simulink model "sgMdl_IO753_IO754_ModbusTCP_Loopback"  (R2024b)
settings: Solver=FixedStepAuto  StartTime=0.0  StopTime=inf  RelTol=1e-3  EnableMultiTasking=on
undefined symbols (not defined in the file): C, IO, Mode, receive_v2, send_v2, setup_v2
libraries: slrealtimeutilitieslib x9, speedgoatlib_IO753 x4, speedgoatlib_IO754 x3, simulink x2
Description:
  | IO753 & IO754 - Modbus TCP Loopback
settings Model: sg_rtwmakecfg_data=_sg_IO75X_v1_2_0__sg_netxLib_MSVC140_  ModifiedByFormat=Speedgoat  SimulationMode=external  ExtModeTrigDuration=100000  Creator=Speedgoat  LastModifiedBy=Speedgoat
settings SolverCC: ConcurrentTasks=on  AlgebraicLoopSolver=TrustRegion  PositivePriorityOrder=on  AutoInsertRateTranBlk=on  InsertRTBMode=Never (minimum delay)
settings DataIOCC: LimitDataPoints=on  SaveFormat=StructureWithTime  ReturnWorkspaceOutputs=off
settings OptimizationCC: BlockReduction=off  BooleanDataType=off  OptimizeBlockIOStorage=off  BufferReuse=off  GlobalBufferReuse=off  ExpressionFolding=off  LocalBlockOutputs=off  OptimizeDataStoreBuffers=off  BusAssignmentInplaceUpdate=off
settings DebuggingCC: SaveWithParameterizedLinksMsg=none  UnderspecifiedInitializationDetection=Classic  MergeDetectMultiDrivingBlocksExec=none  SignalResolutionControl=TryResolveAllWithWarning  InheritedTsInSrcMsg=none  TasksWithSamePriorityMsg=none  ParameterOverflowMsg=none  UnconnectedInputMsg=warning  UnconnectedOutputMsg=warning  UnconnectedLineMsg=warning  SFUnexpectedBacktrackingDiag=warning  SFNoUnconditionalDefaultTransitionDiag=warning  SFExecutionAtInitializationDiag=none  ArithmeticOperatorsInVariantConditions=warning
settings HardwareCC: ProdBitPerLong=64  ProdLongLongMode=on  ProdHWDeviceType=Intel->x86-64 (Linux 64)  TargetBitPerPointer=64  TargetBitPerSizeT=64  TargetBitPerPtrDiffT=64  TargetLongLongMode=on  TargetIntDivRoundTo=Zero  TargetEndianess=LittleEndian  TargetWordSize=64  TargetHWDeviceType=MATLAB Host
settings ModelReferenceCC: EnableRefExpFcnMdlSchedulingChecks=on  PropagateSignalLabelsOutOfModel=off
settings SFSimCC: SimUseLocalCustomCode=off  CustomCodeUndefinedFunction=UseInterfaceOnly
settings RTWCC: Description=Speedgoat Real-Time Target Machine  SystemTargetFile=speedgoat.tlc  TemplateMakefile=slrealtime_default_tmf  RetainRTWFile=on  RTWUseLocalCustomCode=off  Toolchain=Simulink Real-Time Toolchain  BuildConfiguration=Faster Runs  TargetLang=C++  GPUComputeCapability=3.5  DLArmComputeVersion=19.05
settings CodeAppCC: StateflowObjectComments=on
settings SimulinkRealTimeTargetCC: SubcomponentCodeInterfacePackaging=Reusable function  InstructionSetFMA=off  LogToMDFFile=off  SLRTFileLogMaxRuns=10  UseGCCFastMath=on
settings ConfigComp: CovMetricSettings=dw  CovSaveCumulativeToWorkspaceVar=on  CovSaveSingleToWorkspaceVar=on  CovExternalEMLEnable=off  CovBoundaryAbsTol=1.0e-5

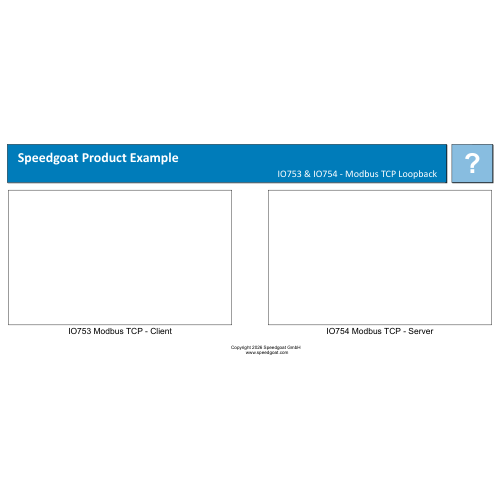
[thumbnail: Simulink's stored preview of the top-level diagram]
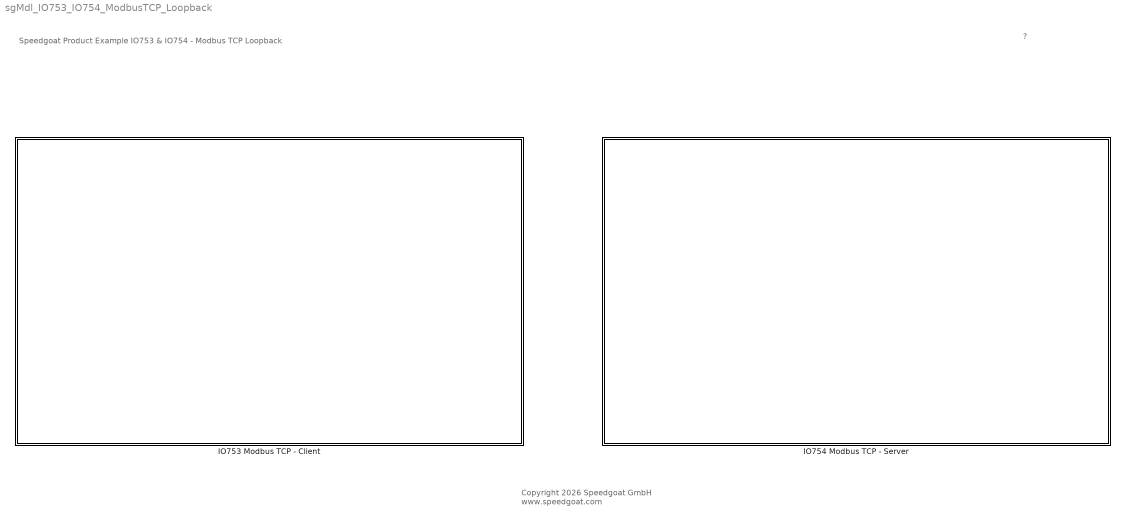
== system sgMdl_IO753_IO754_ModbusTCP_Loopback ==
  note: Speedgoat Product Example
      | IO753 & IO754 - Modbus TCP Loopback
  note: ?
  note: Copyright 2026 Speedgoat GmbH
      |  www.speedgoat.com
  IO753 Modbus TCP - Client : Subsystem
  IO754 Modbus TCP - Server : Subsystem

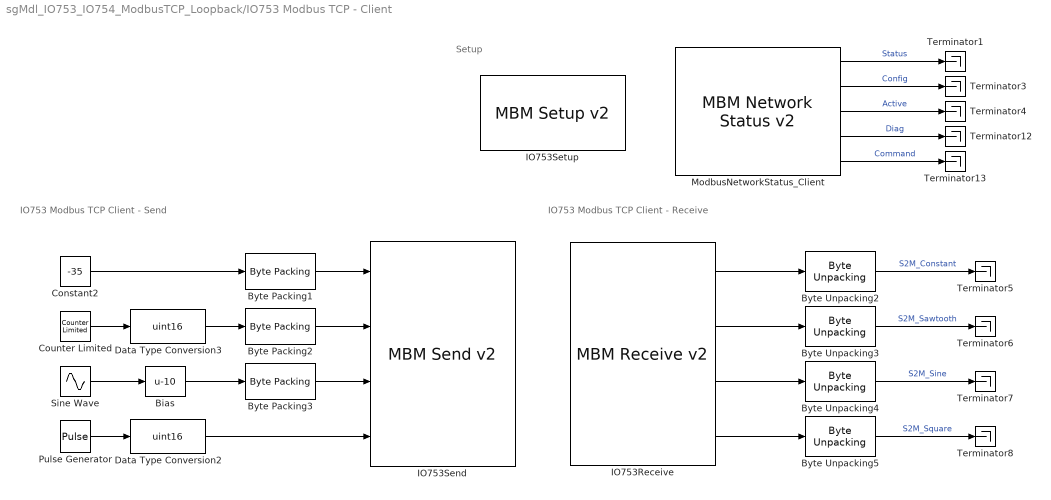
== system sgMdl_IO753_IO754_ModbusTCP_Loopback/IO753 Modbus TCP - Client ==
  note: IO753 Modbus TCP Client - Receive
  note: IO753 Modbus TCP Client - Send
  note: Setup
  Bias : Bias  Bias=-10
  Byte Packing1 : slrealtimeutilitieslib/Byte Packing  MaskPackedDataType=uint16  MaskUnpackedDataTypes={'double'}  MaskAlignment=1
  Byte Packing2 : slrealtimeutilitieslib/Byte Packing  MaskPackedDataType=uint16  MaskUnpackedDataTypes={'uint16'}  MaskAlignment=1
  Byte Packing3 : slrealtimeutilitieslib/Byte Packing  MaskPackedDataType=uint16  MaskUnpackedDataTypes={'double'}  MaskAlignment=1
  Byte Unpacking{2..5} (4 alike) : slrealtimeutilitieslib/Byte Unpacking
  Constant2 : Constant  Value=-35  SampleTime=-1
  Counter Limited : simulink/Sources/Counter Limited  uplimit=53  tsamp=-1
  Data Type Conversion2 : DataTypeConversion  OutMin=[0]  OutMax=[50]  OutDataTypeStr=uint16  SaturateOnIntegerOverflow=off  RndMeth=Floor
  Data Type Conversion3 : DataTypeConversion  OutMin=[0]  OutMax=[100]  OutDataTypeStr=uint16  SaturateOnIntegerOverflow=off  RndMeth=Floor
  IO753Receive : speedgoatlib_IO753/MBM Receive v2  id=1  parSampleTime=-1  parCommandTable={ 'Tx_Constant', 'IP_Server_00', '0', 'FC16 Write Multiple Registers', '0', '4', '50'; 'Tx_Sawtooth', 'IP_Server_00', '0', 'FC6 Write Single Register ', '4', '1', '50'; 'Tx_Sine', 'IP_Server_00', '0', 'FC16 Write Multiple Registers', '5', '4', '50'; 'Tx_Square', 'IP_Server_00', '0', 'FC16 Write Multiple Registers', '9', '1', '50'; 'Rx_Constant', 'IP_Server_00', '0', 'FC3 Read Holding Registers', '0', '1', '50'; 'Rx_Sawtooth', 'IP_Server_00', '0', 'FC3 Read Holding Registers', '1', '1', '50'; 'Rx_Sine', 'IP_Server_00', '0', 'FC3 Read Holding Registers', '2', '4', '50'; 'Rx_Square', 'IP_Server_00', '0', 'FC3 Read Holding Registers', '6', '1', '50' }
      settings: SourceProductName=Simulink Real-Time: Speedgoat I/O Blockset
  IO753Send : speedgoatlib_IO753/MBM Send v2  id=1  parSampleTime=-1  parCommandTable={ 'Tx_Constant', 'IP_Server_00', '0', 'FC16 Write Multiple Registers', '0', '4', '50'; 'Tx_Sawtooth', 'IP_Server_00', '0', 'FC6 Write Single Register ', '4', '1', '50'; 'Tx_Sine', 'IP_Server_00', '0', 'FC16 Write Multiple Registers', '5', '4', '50'; 'Tx_Square', 'IP_Server_00', '0', 'FC16 Write Multiple Registers', '9', '1', '50'; 'Rx_Constant', 'IP_Server_00', '0', 'FC3 Read Holding Registers', '0', '1', '50'; 'Rx_Sawtooth', 'IP_Server_00', '0', 'FC3 Read Holding Registers', '1', '1', '50'; 'Rx_Sine', 'IP_Server_00', '0', 'FC3 Read Holding Registers', '2', '4', '50'; 'Rx_Square', 'IP_Server_00', '0', 'FC3 Read Holding Registers', '6', '1', '50' }
      settings: SourceProductName=Simulink Real-Time: Speedgoat I/O Blockset
  IO753Setup : speedgoatlib_IO753/MBM Setup v2  id=1  parSlot=-1  parBusStart=Automatic  parIpAddress=IP_Client_00  parNetmask='255.255.255.0'  parGateway='0.0.0.0'  parBootP=off  parDHCP=off  DataSwap=off  parDelay=0  parCommandTable={ 'Tx_Constant', 'IP_Server_00', '0', 'FC16 Write Multiple Registers', '0', '4', '50'; 'Tx_Sawtooth', 'IP_Server_00', '0', 'FC6 Write Single Register ', '4', '1', '50'; 'Tx_Sine', 'IP_Server_00', '0', 'FC16 Write Multiple Registers', '5', '4', '50'; 'Tx_Square', 'IP_Server_00', '0', 'FC16 Write Multiple Registers', '9', '1', '50'; 'Rx_Constant', 'IP_Server_00', '0', 'FC3 Read Holding Registers', '0', '1', '50'; 'Rx_Sawtooth', 'IP_Server_00', '0', 'FC3 Read Holding Registers', '1', '1', '50'; 'Rx_Sine', 'IP_Server_00', '0', 'FC3 Read Holding Registers', '2', '4', '50'; 'Rx_Square', 'IP_Server_00', '0', 'FC3 Read Holding Registers', '6', '1', '50' }
      settings: SourceProductName=Simulink Real-Time: Speedgoat I/O Blockset
  ModbusNetworkStatus_Client : speedgoatlib_IO753/MBM Network Status v2  id=1  parSampleTime=-1  parSetStatus=off  parNumServers=0  parNumCommands=0
      settings: SourceProductName=Simulink Real-Time: Speedgoat I/O Blockset
  Pulse Generator : DiscretePulseGenerator  PulseType=Time based  Amplitude=23  Period=3.5  PulseWidth=40  SampleTime=-1
  Sine Wave : Sin  Amplitude=12  Frequency=pi  Phase=pi
  Terminator{1,3..8,12..13} (9 alike) : Terminator
  wires:
  Byte Unpacking4/1 -> Terminator7/1  "S2M_Sine"
  Sine Wave/1 -> Bias/1
  Pulse Generator/1 -> Data Type Conversion2/1
  Byte Unpacking3/1 -> Terminator6/1  "S2M_Sawtooth"
  Byte Unpacking5/1 -> Terminator8/1  "S2M_Square"
  Byte Unpacking2/1 -> Terminator5/1  "S2M_Constant"
  Counter Limited/1 -> Data Type Conversion3/1
  Byte Packing1/1 -> IO753Send/1
  Byte Packing2/1 -> IO753Send/2
  Byte Packing3/1 -> IO753Send/3
  Data Type Conversion2/1 -> IO753Send/4
  IO753Receive/1 -> Byte Unpacking2/1
  IO753Receive/2 -> Byte Unpacking3/1
  IO753Receive/3 -> Byte Unpacking4/1
  IO753Receive/4 -> Byte Unpacking5/1
  ModbusNetworkStatus_Client/2 -> Terminator3/1  "Config"
  ModbusNetworkStatus_Client/1 -> Terminator1/1  "Status"
  ModbusNetworkStatus_Client/3 -> Terminator4/1  "Active"
  ModbusNetworkStatus_Client/4 -> Terminator12/1  "Diag"
  ModbusNetworkStatus_Client/5 -> Terminator13/1  "Command"
  Data Type Conversion3/1 -> Byte Packing2/1
  Bias/1 -> Byte Packing3/1
  Constant2/1 -> Byte Packing1/1

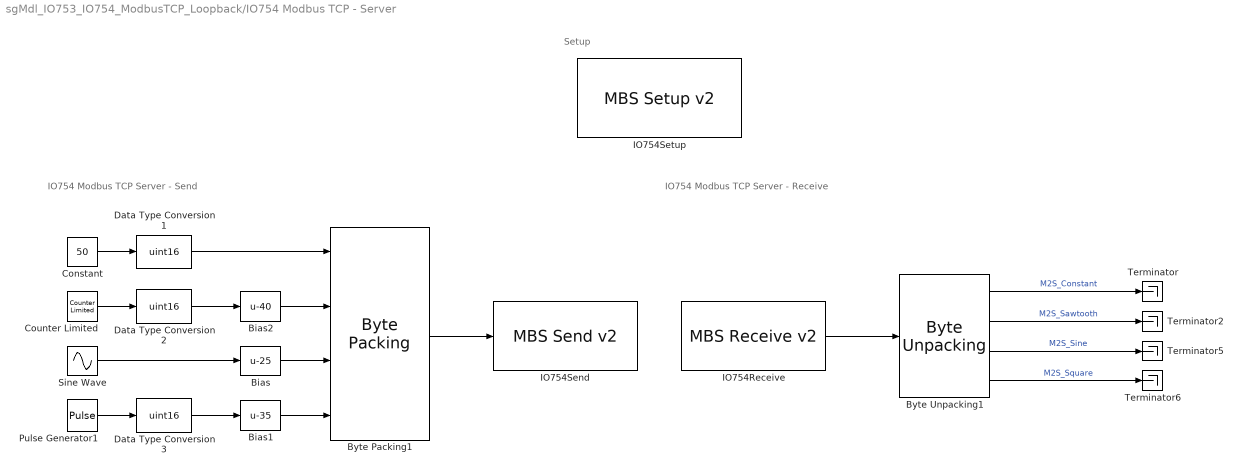
== system sgMdl_IO753_IO754_ModbusTCP_Loopback/IO754 Modbus TCP - Server ==
  note: Setup
  note: IO754 Modbus TCP Server - Send
  note: IO754 Modbus TCP Server - Receive
  Bias : Bias  Bias=-25  SaturateOnIntegerOverflow=off
  Bias1 : Bias  Bias=-35  SaturateOnIntegerOverflow=off
  Bias2 : Bias  Bias=-40  SaturateOnIntegerOverflow=off
  Byte Packing1 : slrealtimeutilitieslib/Byte Packing  MaskPackedDataType=uint8  MaskUnpackedDataTypes={'uint16','uint16','double','uint16'}  MaskAlignment=1
  Byte Unpacking1 : slrealtimeutilitieslib/Byte Unpacking  MaskUnpackedDataTypes={'double','uint16','double','uint16'}  MaskUnpackedDataSizes={[1],[1],[1],[1]}  MaskAlignment=1
  Constant : Constant  Value=50  OutDataTypeStr=Inherit: Inherit via back propagation  SampleTime=-1
  Counter Limited : simulink/Sources/Counter Limited  uplimit=42  tsamp=-1
  Data Type Conversion1 : DataTypeConversion  OutMin=[0]  OutMax=[100]  OutDataTypeStr=uint16  SaturateOnIntegerOverflow=off  RndMeth=Floor
  Data Type Conversion2 : DataTypeConversion  OutMin=[0]  OutMax=[100]  OutDataTypeStr=uint16  SaturateOnIntegerOverflow=off  RndMeth=Floor
  Data Type Conversion3 : DataTypeConversion  OutMin=[0]  OutMax=[50]  OutDataTypeStr=uint16  SaturateOnIntegerOverflow=off  RndMeth=Floor
  IO754Receive : speedgoatlib_IO754/IO-Mode/MBS Receive v2   id=2  portType=1 Port with n element vector of type UINT8  portDataBytes=20  sampleTime=-1  blockInfo=receive_v2;setup_v2  isSender=0  speedgoatMainProtl=IO75X_IO64X  speedgoatSubProtl=IO754
      settings: SourceProductName=Simulink Real-Time: Speedgoat I/O Blockset
  IO754Send : speedgoatlib_IO754/IO-Mode/MBS Send v2   id=2  portType=1 Port with n element vector of type UINT8  portDataBytes=14  sampleTime=-1  blockInfo=send_v2;setup_v2  isSender=1  speedgoatMainProtl=IO75X_IO64X  speedgoatSubProtl=IO754
      settings: SourceProductName=Simulink Real-Time: Speedgoat I/O Blockset
  IO754Setup : speedgoatlib_IO754/MBS Setup v2   id=2  drvLetter=C:  cfgMode=Warmstart  busSlot=-1  opMode=IO-Mode  busStart=Automatic  dataSwap=on  mapFC1FC3=off  serverCon=1  conWdgTime=1000  resTimeout=2000  sndAckTimeout=31000  conAckTimeout=31000  closeAckTimeout=13000  ipAdr=192.168.10.20  netmask='255.255.255.0'  gateway='0.0.0.0'  bootP=off  dhcp=off  enaMsgMode=off  coilStartAdr=0  coilQty=65536  descreteInputsStartAdr=0  descreteInputsQty=65536  holdingRegStartAdr=0  holdingRegQty=65536  inputRegStartAdr=0  inputRegQty=65536  blockInfo=setup_v2  speedgoatMainProtl=IO75X_IO64X  speedgoatSubProtl=IO754  protocolDescirption=Modbus TCP Server (slave)  filesBL="[\"1\", \"NETX100.BIN\"]"  filesFW="[\"1\", \"CIFXOMB.NXF\", \"2.6.0.6\", \"Open Modbus/TCP\"]"  filesCfg="[\"1\", \"INIBATCH.NXD\"]"  devData="[\"0000\", \"15CF\", \"0000\", \"0000\"]"  protocol=IO754  firmware=Modbus TCP Server
      settings: SourceProductName=Simulink Real-Time: Speedgoat I/O Blockset
  Pulse Generator1 : DiscretePulseGenerator  PulseType=Time based  Amplitude=32  Period=3.5  PulseWidth=63  SampleTime=-1
  Sine Wave : Sin  Amplitude=23  Frequency=2*pi  Phase=pi
  Terminator{,2,5..6} (4 alike) : Terminator
  wires:
  Byte Unpacking1/1 -> Terminator/1  "M2S_Constant"
  Byte Packing1/1 -> IO754Send/1
  Byte Unpacking1/3 -> Terminator5/1  "M2S_Sine"
  Byte Unpacking1/2 -> Terminator2/1  "M2S_Sawtooth"
  IO754Receive/1 -> Byte Unpacking1/1
  Byte Unpacking1/4 -> Terminator6/1  "M2S_Square"
  Data Type Conversion3/1 -> Bias1/1
  Constant/1 -> Data Type Conversion1/1
  Data Type Conversion2/1 -> Bias2/1
  Sine Wave/1 -> Bias/1
  Data Type Conversion1/1 -> Byte Packing1/1
  Bias/1 -> Byte Packing1/3
  Pulse Generator1/1 -> Data Type Conversion3/1
  Counter Limited/1 -> Data Type Conversion2/1
  Bias2/1 -> Byte Packing1/2
  Bias1/1 -> Byte Packing1/4
